simulink model "NonLinearHeliGain"  (R2021a)
settings: Solver=VariableStepAuto  StartTime=0.0  StopTime=8.0  MaxStep=1e-3  RelTol=1e-3
values from neighbouring files (symbols this model uses):
  A = [0 0 1 0 ... (first row only)    [HeliControlGain.m]    (also in HeliControlHinf.m; HeliControlInteger.m; HeliControlLQG.m; HeliControlLQRgain.m)
  B = [0 0 ... (first row only)    [HeliControlGain.m]    (also in HeliControlHinf.m; HeliControlInteger.m; HeliControlLQG.m; HeliControlLQRgain.m)
  Bp = 0.8    [HeliControlGain.m]    (also in HeliControlHinf.m; HeliControlInteger.m; HeliControlIntegerObsv.m; HeliControlLQG.m)
  By = 0.318    [HeliControlGain.m]    (also in HeliControlHinf.m; HeliControlInteger.m; HeliControlIntegerObsv.m; HeliControlLQG.m)
  C = [1 0 0 0 ... (first row only)    [HeliControlGain.m]    (also in HeliControlHinf.m; HeliControlInteger.m; HeliControlLQG.m; HeliControlLQRgain.m)
  D = zeros(2,2)    [HeliControlGain.m]    (also in HeliControlHinf.m; HeliControlInteger.m; HeliControlLQG.m; HeliControlLQRgain.m)
  G = Gbar\I    [HeliControlGain.m]    (also in HeliControlHinf.m = ss(A,B,C,D); HeliControlLQRgain.m)
  g = 9.81    [HeliControlGain.m]    (also in HeliControlHinf.m; HeliControlInteger.m; HeliControlIntegerObsv.m; HeliControlLQG.m)
  Jeq_y = 0.0432    [HeliControlGain.m]    (also in HeliControlHinf.m; HeliControlInteger.m; HeliControlIntegerObsv.m; HeliControlLQG.m)
  Jtp = Jeq_p + Mheli*Lcm^2    (= 0.0863915712)    [HeliControlGain.m]    (also in HeliControlHinf.m; HeliControlInteger.m; HeliControlIntegerObsv.m; HeliControlLQG.m)
  K = place(A,B,p)    [HeliControlGain.m]    (also in HeliControlInteger.m = place(Ag,Bg,p); HeliControlIntegerObsv.m = place(Ag,Bg,p); HeliControlLQG.m = lqr(Ag,Bg,Q,R); HeliControlLQRgain.m = lqr(sysHeli,Q,R))
  Kpp = 0.204    [HeliControlGain.m]    (also in HeliControlHinf.m; HeliControlInteger.m; HeliControlIntegerObsv.m; HeliControlLQG.m)
  Kpy = 0.0068    [HeliControlGain.m]    (also in HeliControlHinf.m; HeliControlInteger.m; HeliControlIntegerObsv.m; HeliControlLQG.m)
  Kyp = 0.0219    [HeliControlGain.m]    (also in HeliControlHinf.m; HeliControlInteger.m; HeliControlIntegerObsv.m; HeliControlLQG.m)
  Kyy = 0.072    [HeliControlGain.m]    (also in HeliControlHinf.m; HeliControlInteger.m; HeliControlIntegerObsv.m; HeliControlLQG.m)
  Lcm = 0.186    [HeliControlGain.m]    (also in HeliControlHinf.m; HeliControlInteger.m; HeliControlIntegerObsv.m; HeliControlLQG.m)
  Mheli = 1.3872    [HeliControlGain.m]    (also in HeliControlHinf.m; HeliControlInteger.m; HeliControlIntegerObsv.m; HeliControlLQG.m)
  u0 = a\b    [HeliControlGain.m]    (also in HeliControlHinf.m; HeliControlInteger.m; HeliControlIntegerObsv.m; HeliControlLQG.m)
libraries: simulink x6
settings Model: Creator=Ciro  LastModifiedBy=Ciro
settings SolverCC: AlgebraicLoopSolver=TrustRegion

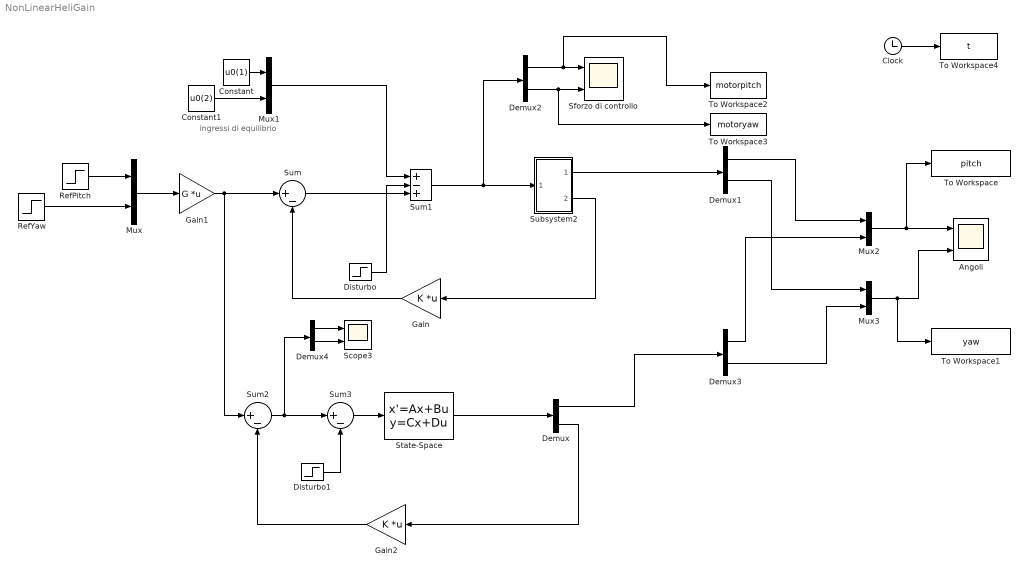
== system NonLinearHeliGain ==
  note: ingressi di equilibrio
  Angoli : Scope  NumInputPorts=2
  Clock : Clock
  Constant : Constant  Value=u0(1)
  Constant1 : Constant  Value=u0(2)
  Demux : Demux  Outputs=[2 4]
  Demux{1..4} (4 alike) : Demux  Outputs=2
  Disturbo : Step  Time=7  After=0  SampleTime=0
  Disturbo1 : Step  Time=7  After=0  SampleTime=0
  Gain : Gain  Gain=K  Multiplication=Matrix(K*u)
  Gain1 : Gain  Gain=G  Multiplication=Matrix(K*u)
  Gain2 : Gain  Gain=K  Multiplication=Matrix(K*u)
  Mux{,1..3} (4 alike) : Mux  Inputs=2
  RefPitch : Step  After=0.3  SampleTime=0
  RefYaw : Step  After=0.3  SampleTime=0
  Scope3 : Scope  NumInputPorts=2
  Sforzo di controllo : Scope  NumInputPorts=2
  State-Space : StateSpace  A=A  B=B  C=[C;eye(4)]  D=[D;zeros(4,2)]  InitialCondition=[0;0;0;0]
  Subsystem2 : Subsystem
  Sum : Sum  Inputs=|+-
  Sum1 : Sum  Inputs=+-+
  Sum2 : Sum  Inputs=|+-
  Sum3 : Sum  Inputs=|+-
  To Workspace : ToWorkspace  VariableName=pitch  SampleTime=-1
      settings: Save2DSignal=2-D array (concatenate along first dimension)
  To Workspace1 : ToWorkspace  VariableName=yaw  SampleTime=-1
      settings: Save2DSignal=2-D array (concatenate along first dimension)
  To Workspace2 : ToWorkspace  VariableName=motorpitch  SampleTime=-1
      settings: Save2DSignal=2-D array (concatenate along first dimension)
  To Workspace3 : ToWorkspace  VariableName=motoryaw  SampleTime=-1
      settings: Save2DSignal=2-D array (concatenate along first dimension)
  To Workspace4 : ToWorkspace  VariableName=t  SampleTime=-1
      settings: Save2DSignal=2-D array (concatenate along first dimension)
  wires:
  RefYaw/1 -> Mux/2
  Gain/1 -> Sum/2
  Mux/1 -> Gain1/1
  Demux2/1 -> To Workspace2/1, Sforzo di controllo/1
  Demux1/2 -> Mux3/1
  RefPitch/1 -> Mux/1
  Demux1/1 -> Mux2/1
  Demux2/2 -> To Workspace3/1, Sforzo di controllo/2
  Constant/1 -> Mux1/1
  Constant1/1 -> Mux1/2
  Gain1/1 -> Sum2/1, Sum/1
  Demux/1 -> Demux3/1
  Sum2/1 -> Sum3/1, Demux4/1
  State-Space/1 -> Demux/1
  Gain2/1 -> Sum2/2
  Demux4/1 -> Scope3/1
  Demux/2 -> Gain2/1
  Demux3/1 -> Mux2/2
  Mux2/1 -> To Workspace/1, Angoli/1
  Demux3/2 -> Mux3/2
  Mux3/1 -> To Workspace1/1, Angoli/2
  Subsystem2/1(Out1) -> Demux1/1
  Subsystem2/2(Out2) -> Gain/1
  Demux4/2 -> Scope3/2
  Sum/1 -> Sum1/3
  Mux1/1 -> Sum1/1
  Sum1/1 -> Subsystem2/1(In1), Demux2/1
  Clock/1 -> To Workspace4/1
  Disturbo/1 -> Sum1/2
  Disturbo1/1 -> Sum3/2
  Sum3/1 -> State-Space/1

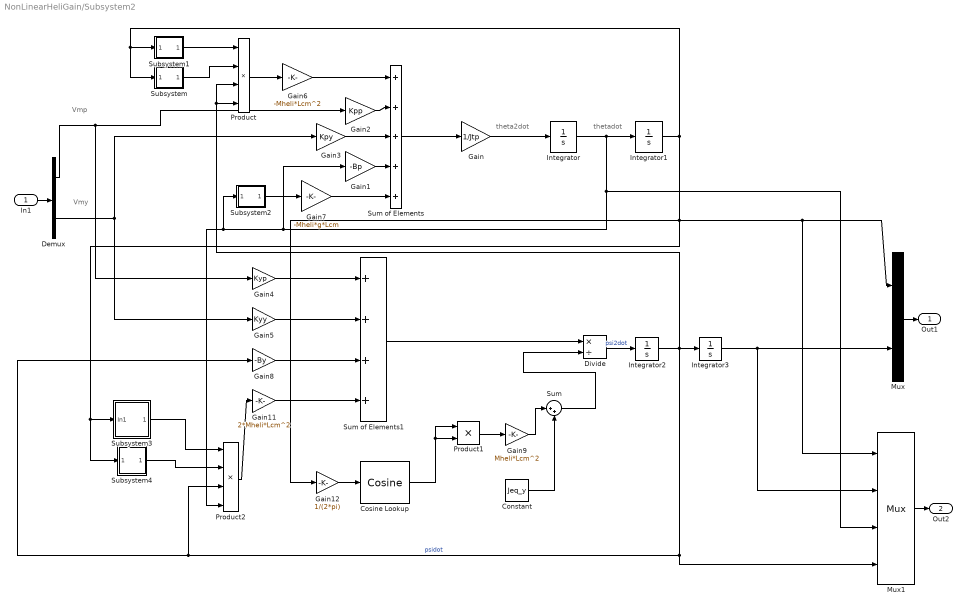
== system NonLinearHeliGain/Subsystem2 ==
  note: theta2dot
  note: thetadot
  note: Vmy
  note: Vmp
  In1 : Inport
  Constant : Constant  Value=Jeq_y
  Cosine Lookup : simulink/Lookup Tables/Cosine  Formula=cos(2*pi*u)  NumDataPoints=(2^5)+1  OutputWordLength=16  InternalRulePriority=Speed
      settings: SourceProductBaseCode=SL
  Demux : Demux  Outputs=2
  Divide : Product  Inputs=*/
  Gain : Gain  Gain=1/Jtp
  Gain1 : Gain  Gain=-Bp
  Gain11 : Gain  Gain=2*Mheli*Lcm^2
  Gain12 : Gain  Gain=1/(2*pi)
  Gain2 : Gain  Gain=Kpp
  Gain3 : Gain  Gain=Kpy
  Gain4 : Gain  Gain=Kyp
  Gain5 : Gain  Gain=Kyy
  Gain6 : Gain  Gain=-Mheli*Lcm^2
  Gain7 : Gain  Gain=-Mheli*g*Lcm
  Gain8 : Gain  Gain=-By
  Gain9 : Gain  Gain=Mheli*Lcm^2
  Integrator{,1..3} (4 alike) : Integrator
  Mux : Mux  Inputs=2
  Mux1 : Mux
  Product : Product  Inputs=4
  Product1 : Product
  Product2 : Product  Inputs=4
  Subsystem : Subsystem
  Subsystem1 : Subsystem
  Subsystem2 : Subsystem
  Subsystem3 : Subsystem
  Subsystem4 : Subsystem
  Sum : Sum  Inputs=|++
  Sum of Elements : Sum  Inputs=+++++
  Sum of Elements1 : Sum  Inputs=++++
  Out1 : Outport
  Out2 : Outport  Port=2
  wires:
  Gain5/1 -> Sum of Elements1/2
  Gain9/1 -> Sum/1
  In1/1 -> Demux/1
  Product1/1 -> Gain9/1
  Subsystem1/1(sin(2*pi*u)) -> Product/1
  Gain3/1 -> Sum of Elements/3
  Gain6/1 -> Sum of Elements/1
  Subsystem/1(cos(2*pi*u)) -> Product/2
  Constant/1 -> Sum/2
  Subsystem4/1(sin(2*pi*u)) -> Product2/2
  Mux1/1 -> Out2/1
  Gain12/1 -> Cosine Lookup/1
  Gain2/1 -> Sum of Elements/2
  Sum of Elements1/1 -> Divide/1
  Cosine Lookup/1 -> Product1/1, Product1/2
  Divide/1 -> Integrator2/1  "psi2dot"
  Gain11/1 -> Sum of Elements1/4
  Mux/1 -> Out1/1
  Gain4/1 -> Sum of Elements1/1
  Gain8/1 -> Sum of Elements1/3
  Product/1 -> Gain6/1
  Gain7/1 -> Sum of Elements/5
  Integrator3/1 -> Mux/2, Mux1/2
  Demux/1 -> Gain2/1, Gain4/1
  Demux/2 -> Gain3/1, Gain5/1
  Subsystem2/1(cos(2*pi*u)) -> Gain7/1
  Integrator2/1 -> Integrator3/1, Product2/3, Gain8/1, Mux1/4, Product/3, Product/4  "psidot"
  Gain/1 -> Integrator/1
  Sum/1 -> Divide/2
  Sum of Elements/1 -> Gain/1
  Gain1/1 -> Sum of Elements/4
  Integrator1/1 -> Subsystem1/1(In1), Subsystem/1(In1), Gain12/1, Mux/1, Mux1/1, Subsystem3/1(In1), Subsystem4/1(In1)
  Product2/1 -> Gain11/1
  Integrator/1 -> Integrator1/1, Subsystem2/1(In1), Product2/4, Gain1/1, Mux1/3
  Subsystem3/1(cos(2*pi*u)) -> Product2/1

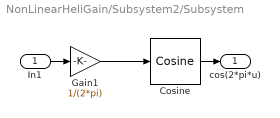
== system NonLinearHeliGain/Subsystem2/Subsystem ==
  In1 : Inport
  Cosine : simulink/Lookup Tables/Cosine  Formula=cos(2*pi*u)  NumDataPoints=(2^5)+1  OutputWordLength=16  InternalRulePriority=Speed
      settings: SourceProductBaseCode=SL
  Gain1 : Gain  Gain=1/(2*pi)
  cos(2*pi*u) : Outport
  wires:
  Cosine/1 -> cos(2*pi*u)/1
  In1/1 -> Gain1/1
  Gain1/1 -> Cosine/1

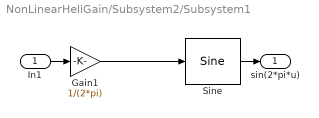
== system NonLinearHeliGain/Subsystem2/Subsystem1 ==
  In1 : Inport
  Gain1 : Gain  Gain=1/(2*pi)
  Sine : simulink/Lookup Tables/Sine  Formula=sin(2*pi*u)  NumDataPoints=(2^5)+1  OutputWordLength=16  InternalRulePriority=Speed
  sin(2*pi*u) : Outport
  wires:
  Sine/1 -> sin(2*pi*u)/1
  In1/1 -> Gain1/1
  Gain1/1 -> Sine/1

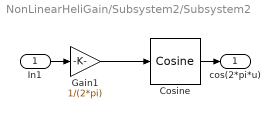
== system NonLinearHeliGain/Subsystem2/Subsystem2 ==
  In1 : Inport
  Cosine : simulink/Lookup Tables/Cosine  Formula=cos(2*pi*u)  NumDataPoints=(2^5)+1  OutputWordLength=16  InternalRulePriority=Speed
      settings: SourceProductBaseCode=SL
  Gain1 : Gain  Gain=1/(2*pi)
  cos(2*pi*u) : Outport
  wires:
  Gain1/1 -> Cosine/1
  In1/1 -> Gain1/1
  Cosine/1 -> cos(2*pi*u)/1

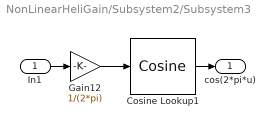
== system NonLinearHeliGain/Subsystem2/Subsystem3 ==
  In1 : Inport
  Cosine Lookup1 : simulink/Lookup Tables/Cosine  Formula=cos(2*pi*u)  NumDataPoints=(2^5)+1  OutputWordLength=16  InternalRulePriority=Speed
      settings: SourceProductBaseCode=SL
  Gain12 : Gain  Gain=1/(2*pi)
  cos(2*pi*u) : Outport
  wires:
  Cosine Lookup1/1 -> cos(2*pi*u)/1
  In1/1 -> Gain12/1
  Gain12/1 -> Cosine Lookup1/1

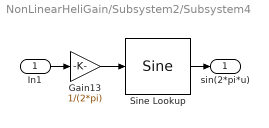
== system NonLinearHeliGain/Subsystem2/Subsystem4 ==
  In1 : Inport
  Gain13 : Gain  Gain=1/(2*pi)
  Sine Lookup : simulink/Lookup Tables/Sine  Formula=sin(2*pi*u)  NumDataPoints=(2^5)+1  OutputWordLength=16  InternalRulePriority=Speed
  sin(2*pi*u) : Outport
  wires:
  In1/1 -> Gain13/1
  Sine Lookup/1 -> sin(2*pi*u)/1
  Gain13/1 -> Sine Lookup/1
